simulink model "current_fed_push_pull_prili"  (R2019a)
settings: Solver=VariableStepAuto  StartTime=0.0  StopTime=Tpwm*30000  RelTol=1e-3
undefined symbols (not defined in the file): Cin, Tpwm, Tss
libraries: powerlib x28, eePwmGenerator x2
settings Model: Creator=asus  LastModifiedBy=asus

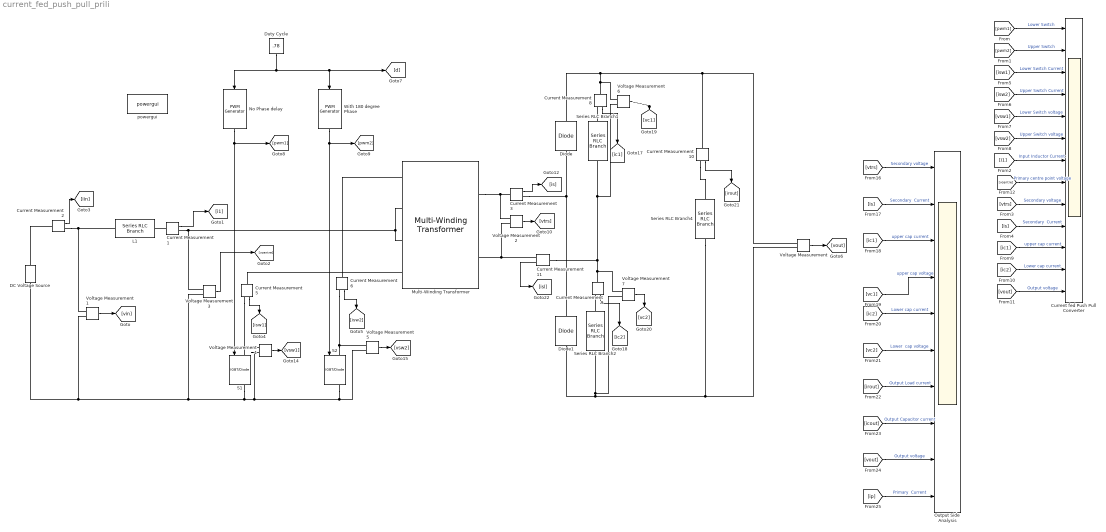
== system current_fed_push_pull_prili ==
  Current Measurement{1..3,5..6,8..11} (9 alike) : powerlib/Measurements/Current Measurement  PhasorSimulation=off  OutputType=Complex  PSBequivalent=0
      settings: SourceProductName=Simscape Electrical
  Current fed Push Pull Converter : Scope  NumInputPorts=13
  DC Voltage Source : powerlib/Electrical Sources/DC Voltage Source  Amplitude=25  Measurements=None
      settings: SourceProductName=Simscape Electrical
  Diode : powerlib/Power Electronics/Diode  Ron=1e-6  Lon=1e-9  Vf=0  IC=0  UseSnubber=0  Rs=500  Cs=250e-9  Measurements=off
      settings: SourceProductName=Simscape Electrical
  Diode1 : powerlib/Power Electronics/Diode  Ron=1e-6  Lon=1e-9  Vf=0  IC=0  UseSnubber=0  Rs=500  Cs=250e-9  Measurements=off
      settings: SourceProductName=Simscape Electrical
  Duty Cycle : Constant  Value=.78
  L1 : powerlib/Elements/Series RLC Branch  LConnTagsString=__new0  RConnTagsString=__new0  BranchType=L  Resistance=1  Inductance=400e-6  SetiL0=off  InitialCurrent=0  Capacitance=Cin  Setx0=off  InitialVoltage=0  Measurements=None
      settings: SourceProductName=Simscape Electrical
  Multi-Winding Transformer : powerlib/Elements/Multi-Winding Transformer  LeftWindings=2  RightWindings=1  TappedWindings=no taps  NumberOfTaps=2  SetSaturation=off  Hysteresis=off  DataFile='hysteresis.mat'  Measurements=None  UNITS=SI  NominalPower=[250 1/Tpwm]  NominalVoltages=[ 100 100 400]  WindingResistances=[0 0 0]  WindingInductances=[0 0 0]  Rm=5.5296e+06  Lm=0.046688  Saturation=[0 0;0.062501 0.029181;26.042 0.036962]  BreakLoop=off  DiscreteSolver=Trapezoidal iterative  DataType=on  InitialFlux=0  TransfoNumber=1
      settings: SourceProductName=Simscape Electrical  SourceProductBaseCode=PS
  No Phase delay : eePwmGenerator/PWM Generator  CarrCount=Up  Tper=Tpwm  Ts=Tss
      settings: SourceProductName=Simscape Electrical
  Output Side Analysis : Scope  NumInputPorts=10
  S1 : powerlib/Power Electronics/IGBT//Diode  Ron=1e-3  Rs=1e5  Cs=inf  Measurements=on
      settings: SourceProductName=Simscape Electrical
  S2 : powerlib/Power Electronics/IGBT//Diode  Ron=1e-3  Rs=1e5  Cs=inf  Measurements=on
      settings: SourceProductName=Simscape Electrical
  Series RLC Branch1 : powerlib/Elements/Series RLC Branch  LConnTagsString=__new0  RConnTagsString=__new0  BranchType=C  Resistance=1  Inductance=1e-3  SetiL0=off  InitialCurrent=0  Capacitance=20e-6  Setx0=off  InitialVoltage=0  Measurements=Branch voltage
      settings: SourceProductName=Simscape Electrical
  Series RLC Branch2 : powerlib/Elements/Series RLC Branch  LConnTagsString=__new0  RConnTagsString=__new0  BranchType=C  Resistance=1  Inductance=1e-3  SetiL0=off  InitialCurrent=0  Capacitance=20e-6  Setx0=off  InitialVoltage=0  Measurements=Branch voltage
      settings: SourceProductName=Simscape Electrical
  Series RLC Branch4 : powerlib/Elements/Series RLC Branch  LConnTagsString=__new0  RConnTagsString=__new0  BranchType=R  Resistance=1000  Inductance=1e-3  SetiL0=off  InitialCurrent=0  Capacitance=470e-6  Setx0=off  InitialVoltage=0  Measurements=None
      settings: SourceProductName=Simscape Electrical
  Voltage Measurement{,1..7} (8 alike) : powerlib/Measurements/Voltage Measurement  PhasorSimulation=off  OutputType=Complex  PSBequivalent=0
      settings: SourceProductName=Simscape Electrical
  With 180 degree Phase : eePwmGenerator/PWM Generator  CarrCount=Up  Tper=Tpwm  Ts=Tss
      link override Carrier counter: Tdelay=Tper*0.5
      settings: SourceProductName=Simscape Electrical
  powergui : powerlib/powergui  Priority=1  SimulationMode=Discrete  SampleTime=Tss  frequency=60  Iterations=50  frequencyindice=0  Pbase=100e6  ErrMax=1e-4  UnitsV=kV  UnitsW=MW  buscounter=0  FunctionMessages=off  echomessages=off  EnableUseOfTLC=off  CurrentSourceSwitches=off  DisableSnubberDevices=off  DisableRonSwitches=off  DisableVfSwitches=off  DisplayEquations=off  AutomaticDiscreteSolvers=off  SolverType=Tustin/Backward Euler (TBE)  Interpol=off  ExternalGateDelay=off  methode=off  Ts=100  x0status=blocks  SPID=on  SwTol=0  HookPort=off  NonlinearTolerance=0  nMaxIteration=15  ContinueOnMaxIteration=off  RestoreLinks=warning  ResistiveCurrentMeasurement=off  Frange=[0:2:500]  Ylog=off  Xlog=on  ShowGrid=off  save=off  variable=ZData  structure=0  ZoomFFT=off  StartTime=0.0  cycles=1  DisplayStyle=1  fundamental=60  FreqAxis=off  MaxFrequency=1000  frequencyindicesteady=1  RmsSteady=1  display=off
      settings: SourceProductName=Simscape Electrical
  wires:
  Voltage Measurement6/1 -> [vc1]
  [ip] -> Output Side Analysis/10  "Primary  Current"
  [icout] -> Output Side Analysis/8  "Output Capacitor current"
  [irout] -> Output Side Analysis/7  "Output Load current"
  Voltage Measurement5/1 -> [vsw2]
  [isw2] -> Current fed Push Pull Converter/4  "Upper Switch Current"
  Voltage Measurement1/1 -> [vin]
  With 180 degree Phase/1 -> S2/1, [pwm2]
  Current Measurement1/1 -> [i1]
  No Phase delay/1 -> [pwm1], S1/1
  Voltage Measurement2/1 -> [vtrs]
  Current Measurement3/1 -> [is]
  Current Measurement2/1 -> [iin]
  Voltage Measurement7/1 -> [vc2]
  [ic2] -> Output Side Analysis/5  "Lower cap current"
  Current Measurement10/1 -> [irout]
  [vc2] -> Output Side Analysis/6  "Lower  cap voltage"
  Current Measurement9/1 -> [ic2]
  [vsw1] -> Current fed Push Pull Converter/5  "Lower Switch voltage"
  Voltage Measurement4/1 -> [vsw1]
  Current Measurement8/1 -> [ic1]
  [i1] -> Current fed Push Pull Converter/7  "Input Inductor Current"
  [is] -> Output Side Analysis/2  "Secondary  Current"
  [pwm2] -> Current fed Push Pull Converter/2  "Upper Switch"
  Duty Cycle/1 -> No Phase delay/1, [d], With 180 degree Phase/1
  Voltage Measurement/1 -> [vout]
  [vout] -> Output Side Analysis/9  "Output voltage"
  Current Measurement11/1 -> [isl]
  [vtrs] -> Output Side Analysis/1  "Secondary voltage"
  Current Measurement5/1 -> [isw1]
  [vsw2] -> Current fed Push Pull Converter/6  "Upper Switch voltage"
  [pwm1] -> Current fed Push Pull Converter/1  "Lower Switch"
  [isw1] -> Current fed Push Pull Converter/3  "Lower Switch Current"
  Current Measurement6/1 -> [isw2]
  [ic1] -> Output Side Analysis/3  "upper cap current"
  [vc1] -> Output Side Analysis/4  "upper cap voltage"
  Voltage Measurement3/1 -> [vcentre]
  [vcentre] -> Current fed Push Pull Converter/8  "Primary centre point voltage"
  [vtrs] -> Current fed Push Pull Converter/9  "Secondary voltage"
  [is] -> Current fed Push Pull Converter/10  "Secondary  Current"
  [ic1] -> Current fed Push Pull Converter/11  "upper cap current"
  [ic2] -> Current fed Push Pull Converter/12  "Lower cap current"
  [vout] -> Current fed Push Pull Converter/13  "Output voltage"
  connections:
  Current Measurement3/RConn1 -- Diode/LConn1 -- Diode1/RConn1
  S1/LConn1 -- Voltage Measurement4/LConn1 -- Current Measurement5/RConn1
  Voltage Measurement/LConn2 -- Diode1/LConn1 -- Series RLC Branch2/RConn1 -- Voltage Measurement7/LConn2 -- Series RLC Branch4/RConn1
  Voltage Measurement1/LConn1 -- L1/LConn1 -- Current Measurement2/RConn1
  Current Measurement9/LConn1 -- Voltage Measurement7/LConn1 -- Current Measurement11/LConn1 -- Voltage Measurement6/LConn2 -- Series RLC Branch1/RConn1
  S1/RConn1 -- DC Voltage Source/LConn1 -- Voltage Measurement1/LConn2 -- Voltage Measurement3/LConn2 -- S2/RConn1 -- Voltage Measurement5/LConn2 -- Voltage Measurement4/LConn2
  Current Measurement8/LConn1 -- Current Measurement10/LConn1 -- Voltage Measurement/LConn1 -- Diode/RConn1 -- Voltage Measurement6/LConn1
  Voltage Measurement2/LConn2 -- Current Measurement11/RConn1 -- Multi-Winding Transformer/RConn2
  S2/LConn1 -- Current Measurement6/RConn1 -- Voltage Measurement5/LConn1
  Current Measurement3/LConn1 -- Voltage Measurement2/LConn1 -- Multi-Winding Transformer/RConn1
  Current Measurement2/LConn1 -- DC Voltage Source/RConn1
  Series RLC Branch1/LConn1 -- Current Measurement8/RConn1
  Current Measurement1/LConn1 -- L1/RConn1
  Current Measurement10/RConn1 -- Series RLC Branch4/LConn1
  Series RLC Branch2/LConn1 -- Current Measurement9/RConn1
  Multi-Winding Transformer/LConn2 -- Voltage Measurement3/LConn1 -- Current Measurement1/RConn1 -- Multi-Winding Transformer/LConn3
  Current Measurement5/LConn1 -- Multi-Winding Transformer/LConn4
  Current Measurement6/LConn1 -- Multi-Winding Transformer/LConn1
